simulink model "A3_FromStartToGoal"  (R2022a)
settings: Solver=FixedStepAuto  StartTime=0.0  StopTime=inf  FixedStep=0.1  RelTol=1e-3
values from neighbouring files (symbols this model uses):
  pathAng = [path thV]    [A2_PathDefinition.m]
undefined symbols (not defined in the file or in its folder): Angular, Linear
libraries: robotlib x4
settings Model: Creator=jacopo  LastModifiedBy=jacopo
settings OptimizationCC: EnhancedBackFolding=on  PassReuseOutputArgsAs=Individual arguments  ZeroExternalMemoryAtStartup=off  ZeroInternalMemoryAtStartup=off  MaxStackSize=64  OptimizeBlockOrder=speed  DifferentSizesBufferReuse=on  OptimizationCustomize=off  EfficientTunableParamExpr=on
settings DebuggingCC: ParameterTunabilityLossMsg=error
settings HardwareCC: ProdBitPerPointer=32  ProdBitPerSizeT=32  ProdBitPerPtrDiffT=32  ProdLargestAtomicFloat=None  ProdIntDivRoundTo=Undefined  ProdEndianess=Unspecified  ProdWordSize=32  ProdHWDeviceType=Generic->Unspecified (assume 32-bit Generic)
settings SFSimCC: MATLABDynamicMemAlloc=off
settings RTWCC: SystemTargetFile=ert.tlc  HardwareBoard=Robot Operating System (ROS)  TLCOptions="-aInlineSetEventsForThisBaseRateFcn=TLC_FALSE -aSuppressMultiTaskScheduler=TLC_FALSE  -aRateBasedStepFcn=0"  TemplateMakefile=ert_default_tmf  Toolchain=Catkin  TargetLang=C++
settings CodeAppCC: ForceParamTrailComments=on  IgnoreCustomStorageClasses=off  OperatorAnnotations=on  SimulinkDataObjDesc=on  SFDataObjDesc=on  InsertBlockDesc=on

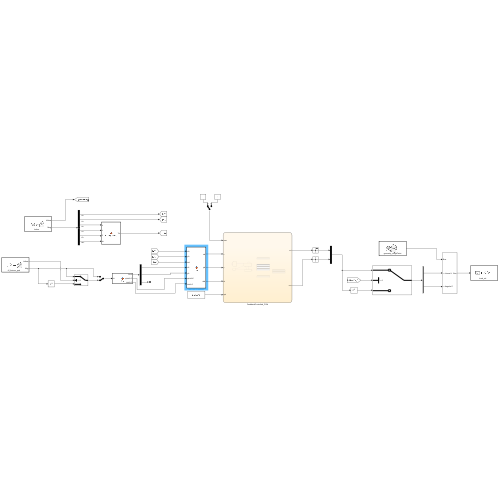
[thumbnail: Simulink's stored preview of the top-level diagram]
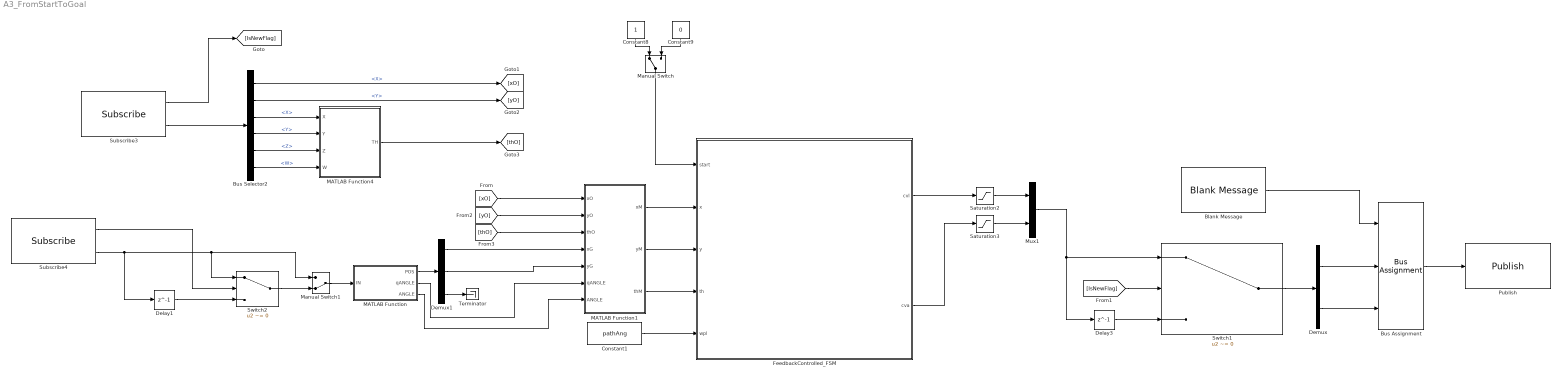
== system A3_FromStartToGoal ==
  Blank Message : robotlib/Blank Message  messageClass=Message  entityType=geometry_msgs/Twist  messageType=geometry_msgs/Twist  SampleTime=inf  legacyBusStruct=off
  Bus Assignment : BusAssignment  AssignedSignals=Linear.X,Angular.Z
  Bus Selector2 : BusSelector  OutputSignals=Pose.Pose.Position.X,Pose.Pose.Position.Y,Pose.Pose.Orientation.X,Pose.Pose.Orientation.Y,Pose.Pose.Orientation.Z,Pose.Pose.Orientation.W
  Constant1 : Constant  Value=pathAng
  Constant8 : Constant
  Constant9 : Constant  Value=0
  Delay1 : Delay  DelayLength=1
  Delay3 : Delay  DelayLength=1
  Demux : Demux  Outputs=2
  Demux1 : Demux  Outputs=3
  FeedbackControlled_FSM : Stateflow chart  TreatAsAtomicUnit=on
  MATLAB Function : MATLAB Function  TreatAsAtomicUnit=on
  MATLAB Function1 : MATLAB Function  TreatAsAtomicUnit=on
  MATLAB Function4 : MATLAB Function  TreatAsAtomicUnit=on
  Manual Switch : ManualSwitch
  Manual Switch1 : ManualSwitch  CurrentSetting=0
  Mux1 : Mux  Inputs=2
  Publish : robotlib/Publish  topicSource=Select from ROS network  topic=/cmd_vel  messageType=geometry_msgs/Twist  legacyBusStruct=off  messageQueueLength=1
  Saturation2 : Saturate  UpperLimit=0.2  LowerLimit=-0.2
  Saturation3 : Saturate  UpperLimit=0.4  LowerLimit=-0.4
  Subscribe3 : robotlib/Subscribe  topicSource=Select from ROS network  topic=/odom  messageType=nav_msgs/Odometry  SampleTime=-1  legacyBusStruct=off  messageQueueLength=1
  Subscribe4 : robotlib/Subscribe  topicSource=Select from ROS network  topic=/tf_listener_pub  messageType=geometry_msgs/PoseWithCovariance  SampleTime=-1  legacyBusStruct=off  messageQueueLength=1
  Switch1 : Switch  Criteria=u2 ~= 0  SaturateOnIntegerOverflow=off  InputSameDT=off
  Switch2 : Switch  Criteria=u2 ~= 0  SaturateOnIntegerOverflow=off  InputSameDT=off
  Terminator : Terminator
  wires:
  Blank Message/1 -> Bus Assignment/1
  Bus Assignment/1 -> Publish/1
  Demux/1 -> Bus Assignment/2
  Demux/2 -> Bus Assignment/3
  Switch1/1 -> Demux/1
  [IsNewFlag] -> Switch1/2
  Delay3/1 -> Switch1/3
  Mux1/1 -> Delay3/1, Switch1/1
  Subscribe3/1 -> [IsNewFlag]
  Bus Selector2/5 -> MATLAB Function4/3(Z)  "<Z>"
  Bus Selector2/3 -> MATLAB Function4/1(X)  "<X>"
  Subscribe3/2 -> Bus Selector2/1
  Bus Selector2/4 -> MATLAB Function4/2(Y)  "<Y>"
  Bus Selector2/1 -> [xO]  "<X>"
  MATLAB Function4/1(TH) -> [thO]
  Bus Selector2/2 -> [yO]  "<Y>"
  Constant9/1 -> Manual Switch/2
  Manual Switch/1 -> FeedbackControlled_FSM/1(start)
  Constant8/1 -> Manual Switch/1
  Saturation2/1 -> Mux1/1
  FeedbackControlled_FSM/1(cvl) -> Saturation2/1
  Saturation3/1 -> Mux1/2
  FeedbackControlled_FSM/2(cva) -> Saturation3/1
  Constant1/1 -> FeedbackControlled_FSM/5(wpl)
  Bus Selector2/6 -> MATLAB Function4/4(W)  "<W>"
  MATLAB Function/1(POS) -> Demux1/1
  Demux1/3 -> Terminator/1
  [xO] -> MATLAB Function1/1(xO)
  [yO] -> MATLAB Function1/2(yO)
  [thO] -> MATLAB Function1/3(thO)
  Demux1/1 -> MATLAB Function1/4(xG)
  Demux1/2 -> MATLAB Function1/5(yG)
  MATLAB Function1/3(thM) -> FeedbackControlled_FSM/4(th)
  MATLAB Function1/2(yM) -> FeedbackControlled_FSM/3(y)
  MATLAB Function1/1(xM) -> FeedbackControlled_FSM/2(x)
  MATLAB Function/2(qANGLE) -> MATLAB Function1/6(qANGLE)
  MATLAB Function/3(ANGLE) -> MATLAB Function1/7(ANGLE)
  Subscribe4/1 -> Switch2/2
  Delay1/1 -> Switch2/3
  Subscribe4/2 -> Delay1/1, Manual Switch1/1, Switch2/1
  Switch2/1 -> Manual Switch1/2
  Manual Switch1/1 -> MATLAB Function/1(IN)

== matlab function A3_FromStartToGoal/MATLAB Function1 ==
  data: xO input; xM output; yO input; thO input; xG input; yG input; yM output; thM output; qANGLE input; ANGLE input
function [xM, yM, thM] = fcn(xO, yO, thO, xG, yG, qANGLE, ANGLE)

swV = 1;

if swV == 0
%   hp: same orientation
    xM = xG + xO;
    yM = yG + yO;
    thM = thO;

elseif swV == 1
%   hp: simplified different orientation
    R = quat2rotm(qANGLE);
    
    tmp = R(1:2, 1:2)*[xO; yO];
    xOp = tmp(1);
    yOp = tmp(2);
    
    xM = xG + xOp;
    yM = yG + yOp;
    thM = thO + ANGLE(1);
elseif swV == 2
%   hp: complex different orientation
%   can't run here: don't have extracted zO and zG 
    R = quat2rotm(qANGLE);
    A = [R [xG; yG; zG]; zeros(1, 3) 1];
    z = [xO; yO; zO];
    x = A*z;
    xM = x(1);
    yM = x(2);
end

end

== matlab function A3_FromStartToGoal/MATLAB Function ==
  data: IN input; POS output; qANGLE output; ANGLE output
function [POS, qANGLE, ANGLE]  =  fcn(IN)

u = IN.Covariance;

x = -u(1);
y = -u(2);
z = -u(3);

X = -u(4);
Y = -u(5);
Z = -u(6);
W =  u(7);

POS = [x, y, z];
qANGLE =  [W, X, Y, Z];
ANGLE = quat2eul(qANGLE);


end

== stateflow chart A3_FromStartToGoal/FeedbackControlled_FSM ==
  state Still
    cvl = 0;
    cva = 0;
    index = 1;
    kPL = 0.5;
    kPA = 2.2;
    overT = 1;
    Dist = 0;
    ErrTh = 0;
    sDSw = 0;
    cvlFix = 0;
    SW = 0;
    Tc =0;
  state FBMotion
    [Dist, ErrTh] = disterrfun(x, y, th, wpl, index);
    [cvl, SW] = cvlCalc(Dist, index, wpl, cvl, Tc, SW, ErrTh);
    cva = cvaCalc(ErrTh);
  state Stop
    cvl = 0;
    cva = 0;
  state Turning
    [Dist, ErrTh] = disterrfun(x, y, th, wpl, index);
    cvl = cvlFix;
    cva = (1*kPA)*ErrTh;
  (default) -> Still
  FBMotion -> FBMotion [order 2] : [Dist > 0.1]{Tc = elapsed(sec)}
  Still -> Still [order 1] : [start == 0]
  Still -> FBMotion [order 2] : [start == 1]
  FBMotion -> Stop [order 1] : [index == length(wpl) + 1]
  Turning -> FBMotion [order 3] : [abs(ErrTh) <= 0.2] {index = index + 1}
  FBMotion -> Turning [order 3] : [Dist <= 0.1] {cvlFix = cvl, SW = 0}
  Turning -> Stop [order 1] : [abs(ErrTh)  <= 0.2 && index == length(wpl)]
  Turning -> Turning [order 2] : [abs(ErrTh) > 0.2]{Tc = elapsed(sec)}
  data: X function_input; Y function_input; Th function_input; WPL function_input; dist function_output; errTh function_output; IND function_input; dist function_input; CVL function_output; ind function_input; WPL function_input; CVLin function_input; tC function_input; sw function_input; swout function_output; th function_input; ETH function_input; CVA function_output; start input; x input; y input; th input; wpl input; Dist local; ErrTh local; cvl output; cva output; index local; kPA local; kPL local; overT local; sDSw local; Tc local; SW local; cvlFix local
  function [dist, errTh] = disterrfun(X, Y, Th, WPL, IND):
    | function [dist, errTh] = disterrfun(X, Y, Th, WPL, IND)
    |  
    | tol = 1e-2;
    | 
    | POSr = WPL(IND, :);
    | 
    | Xr = POSr(1);
    | Yr = POSr(2);
    | Thr = POSr(3);
    | 
    | Gr = Thr;
    | 
    | Z = (Xr - X) + 1i*(Yr - Y);
    | dist = abs(Z);
    | 
    | if dist <= 0.2
    |     if (Th > tol) && (- pi + tol < Gr && Gr < - pi/2 - tol)
    |         Gr = Gr + 2*pi;
    |     elseif (- pi + tol < Th && Th < - pi/2 - tol) && (Gr > tol)
    |         Th = Th + 2*pi;
    |     end
    | else
    |     Gr = angle(Z);
    | 
    |     if (Th > tol) && (- pi + tol < Gr && Gr < - pi/2 - tol)
    |         Gr = Gr + 2*pi;
    |     elseif (- pi + tol < Th && Th < - pi/2 - tol) && (Gr > tol)
    |         Th = Th + 2*pi;
    |     end
    | 
    | 
    | end
    | 
    | 
    | errTh = Gr - Th;
  function [CVL, swout]  = cvlCalc(dist, ind, WPL, CVLin, tC, sw, th):
    | function [CVL, swout]  = cvlCalc(dist, ind, WPL, CVLin, tC, sw, th)
    | 
    | persistent a
    | 
    | C = 1.25;
    | kR1 = 0.1;
    | kR2 = 0.5;
    | 
    | a3 = 0.005;
    | 
    | cvlTh = 0.08;
    | 
    | TH = WPL(ind, 3);
    | 
    | if dist <= 0.5 && sw == 0
    | % this part calculates the deceleration 
    | 	cvlin0 = CVLin;
    |     if 1e-2 - pi/2 < abs(TH - th) && abs(TH - th) < pi + 1e-2
    |         a = ((kR1*cvlin0)^2 - cvlin0^2)*C;
    |         a = 5*a;
    |     else
    |         a = ((kR2*cvlin0)^2 - cvlin0^2)*C;
    |     end
    |     swout = 1;
    | else
    |     a = 0;
    |     swout = 0;
    | end
    | 
    | if dist <= 0.5
    |     CVL = CVLin + a*tC;
    | else
    | 
    |     cvlTmp = CVLin + a3;
    |     CVL = (cvlTmp)*(cvlTmp <= 0.2) + (0.2)*(cvlTmp > 0.2);
    | 
    | end
    | 
    | CVL = CVL*(CVL >= cvlTh) + cvlTh*(CVL < cvlTh);
    | 
    | end
  function CVA = cvaCalc(ETH):
    | function CVA = cvaCalc(ETH)
    | 
    | k1 = 1.8;
    | k2 = 0.8;
    | 
    | tol = 90 * pi/180;
    | 
    | if abs(ETH) > tol
    |     CVA = k1*ETH;
    | else
    |     CVA = k2*ETH;
    | end

== matlab function A3_FromStartToGoal/MATLAB Function4 ==
  data: X input; TH output; Y input; Z input; W input
function TH = fromQuat2Eu(X, Y, Z, W)

ANGLE = quat2eul([W, X, Y, Z]);

TH = ANGLE(1);
